simulink model "GenOptRockerMomtryDisHndlr_harness"  (R2017b)
settings: Solver=FixedStepDiscrete  StartTime=0.0  StopTime=0.9  FixedStep=SAMPLE_TIME_CONFIGSET_0p01_S  RelTol=1e-3
undefined symbols (not defined in the file or in its folder): EnCtrlDisSt, EnCtrlSeln, EnCtrlSts, sigbuilder_block
libraries: simulink x1
settings Model: SldvGeneratedHarnessModel=TestUnitModel=temp_GenOptRockerMomtryDisHndlr|  Creator=KIH3CPW  LastModifiedBy=KIH3CPW
settings DataIOCC: SaveOutput=off  SaveTime=off
settings OptimizationCC: DefaultParameterBehavior=Inlined  ZeroExternalMemoryAtStartup=off  ZeroInternalMemoryAtStartup=off  NoFixptDivByZeroProtection=on  EfficientFloat2IntCast=on  LifeSpan=inf
settings DebuggingCC: SignalInfNanChecking=error  SignalRangeChecking=warning  AlgebraicLoopMsg=error  SaveWithDisabledLinksMsg=error  SaveWithParameterizedLinksMsg=error  BlockPriorityViolationMsg=error  SolverPrmCheckMsg=warning  InheritedTsInSrcMsg=none  CheckMatrixSingularityMsg=error  IntegerOverflowMsg=error  ParameterUnderflowMsg=error  ParameterTunabilityLossMsg=error  FixptConstUnderflowMsg=warning  FixptConstOverflowMsg=error  VectorMatrixConversionMsg=warning  SignalLabelMismatchMsg=warning  UnconnectedInputMsg=error  UnconnectedOutputMsg=error  UnconnectedLineMsg=error  SFcnCompatibilityMsg=warning  FrameProcessingCompatibilityMsg=warning  UniqueDataStoreMsg=error  RootOutportRequireBusObject=error  AssertControl=DisableAll  ModelReferenceIOMismatchMessage=warning  UnknownTsInhSupMsg=error  StateNameClashWarn=warning  StrictBusMsg=ErrorOnBusTreatedAsVector  NonBusSignalsTreatedAsBus=warning  IntegerSaturationMsg=error
settings HardwareCC: ProdBitPerPointer=32  ProdBitPerSizeT=32  ProdBitPerPtrDiffT=32  ProdLargestAtomicInteger=Long  ProdLargestAtomicFloat=Double  ProdEndianess=BigEndian  ProdWordSize=32  ProdHWDeviceType=Freescale->32-bit PowerPC
settings ModelReferenceCC: EnableRefExpFcnMdlSchedulingChecks=off  ModelReferencePassRootInputsByReference=off
settings SFSimCC: SimGenImportedTypeDefs=on  MATLABDynamicMemAlloc=off
settings RTWCC: SystemTargetFile=autosar.tlc  GenCodeOnly=on  TemplateMakefile=ert_default_tmf  Description=AUTOSAR  GenerateReport=on  IncludeHyperlinkInReport=on  LaunchReport=on  GenerateTraceInfo=on  GenerateTraceReport=on  GenerateTraceReportSl=on  GenerateTraceReportSf=on  GenerateTraceReportEml=on
settings CodeAppCC: IgnoreCustomStorageClasses=off  MaxIdLength=63  SimulinkDataObjDesc=on  SFDataObjDesc=on  InsertBlockDesc=on  StateflowObjectComments=on  MATLABSourceComments=on
settings STFCustomTargetCC: TargetLangStandard=C99 (ISO)  CodeReplacementLibrary=JD IFL IFX CRL Tables  MultiwordLength=256  ParMdlRefBuildCompliant=on  CompOptLevelCompliant=on  IncludeMdlTerminateFcn=off  CombineOutputUpdateFcns=on  SuppressErrorStatus=on  ERTCustomFileBanners=on  MultiInstanceERTCode=on  CodeInterfacePackaging=Reusable function  SupportNonFinite=off  SupportComplex=off  SupportContinuousTime=off  SupportNonInlinedSFcns=off  RemoveResetFunc=on  ParenthesesLevel=Maximum  MATLABClassNameForMDSCustomization=Simulink.SoftwareTarget.ERTCustomization  AutosarCompliant=on  GRTInterface=off  UseToolchainInfoCompliant=on  LookupTableObjectStructAxisOrder=2,1,3,4,...  LUTObjectStructOrderEvenSpacing=Size,Table,Breakpoints  SystemTargetFile=autosar.tlc
settings ERTTargetCC: TargetLangStandard=C99 (ISO)  CodeReplacementLibrary=JD IFL IFX CRL Tables  ConcurrentExecutionCompliant=off  IncludeMdlTerminateFcn=off  SuppressErrorStatus=on  MultiInstanceERTCode=on  CodeInterfacePackaging=Reusable function  SupportNonFinite=off  SupportComplex=off  ParenthesesLevel=Maximum  ModelStepFunctionPrototypeControlCompliant=off  CPPClassGenCompliant=off  AutosarCompliant=on  LookupTableObjectStructAxisOrder=2,1,3,4,...  LUTObjectStructOrderEvenSpacing=Size,Table,Breakpoints  InlinedParameterPlacement=NonHierarchical  ERTSrcFileBannerTemplate=JD_AUTOSAR_ert_code_template.cgt  ERTHdrFileBannerTemplate=JD_AUTOSAR_ert_code_template.cgt  ERTDataSrcFileTemplate=JD_AUTOSAR_ert_code_template.cgt  ERTDataHdrFileTemplate=JD_AUTOSAR_ert_code_template.cgt  ERTCustomFileTemplate=example_file_process.tlc
settings ConfigComp: CovEnable=on  RecordCoverage=on  CovSaveName=cvdata  CovMetricSettings=dcmw  CovHTMLOptions=on  CovHtmlReporting=on  CovSaveCumulativeToWorkspaceVar=on  CovSaveSingleToWorkspaceVar=on  CovCumulativeReport=on  CovShowResultsExplorer=off  CovReportOnPause=off  CovModelRefEnable=on

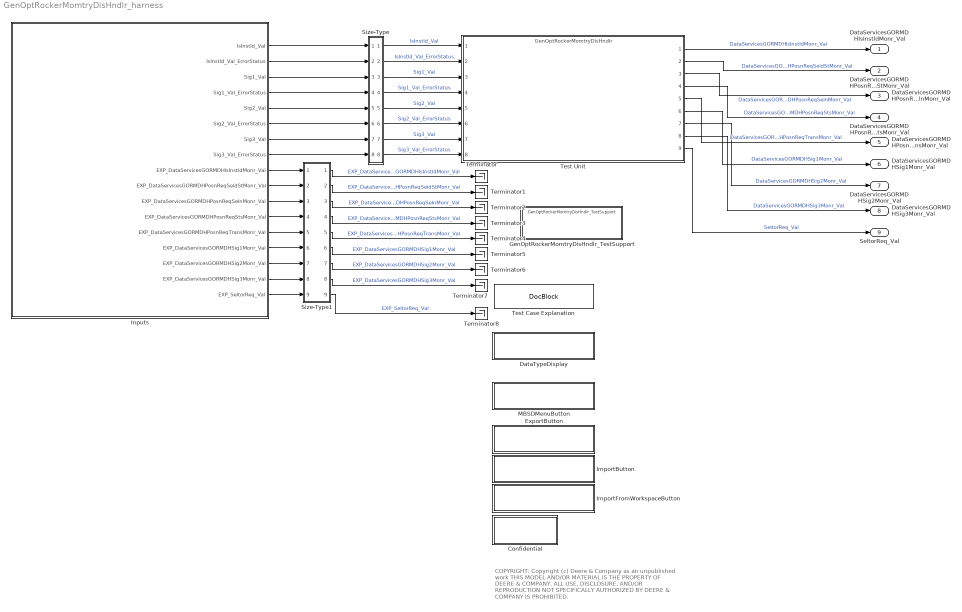
== system GenOptRockerMomtryDisHndlr_harness ==
  note: COPYRIGHT:
      | Copyright (c) Deere & Company as an unpublished work
      | THIS MODEL AND/OR MATERIAL IS THE PROPERTY OF
      | DEERE & COMPANY.  ALL USE, DISCLOSURE, AND/OR
      | REPRODUCTION NOT SPECIFICALLY AUTHORIZED BY
      | DEERE & COMPANY IS PROHIBITED.
  Confidential : Subsystem
      mask Display: image('ConfidentialStamp.jpg')
  DataTypeDisplay : Subsystem  LoadFcn=set_param(gcb,'AttributesFormatString','');  StartFcn=set_param(gcb,'AttributesFormatString','');
      settings: OpenFcn=set_param(gcb,'AttributesFormatString',findModelIDT(gcs));
      mask Display: fprintf(['Double-click to show' char(10) 'Base Data Type'])
  ExportButton : Subsystem  LoadFcn=set_param(gcb,'AttributesFormatString','');  StartFcn=set_param(gcb,'AttributesFormatString','');
      settings: OpenFcn=JD.Model.AddImportExportSwitch.PerformExport(gcs)
      mask Display: fprintf(['Export Data from Signal Builder'])
  GenOptRockerMomtryDisHndlr_TestSupport : ModelReference  ModelNameDialog=GenOptRockerMomtryDisHndlr_TestSupport  SimulationMode=Normal  ModelReferenceVersion=1.1
  ImportButton : Subsystem  LoadFcn=set_param(gcb,'AttributesFormatString','');  StartFcn=set_param(gcb,'AttributesFormatString','');
      settings: OpenFcn=JD.Model.AddImportExportSwitch.PerformImport(gcs)
      mask Display: fprintf(['Import Data to Signal Builder'])
  ImportFromWorkspaceButton : Subsystem  LoadFcn=set_param(gcb,'AttributesFormatString','');  StartFcn=set_param(gcb,'AttributesFormatString','');
      settings: OpenFcn=JD.Model.AddImportExportSwitch.PerformImportfromWorkspace(gcs)
      mask Display: fprintf(['Import Data from Workspace'])
  Inputs : Subsystem  Tag=STV Subsys  LoadFcn=sigbuilder_block('load');  StartFcn=sigbuilder_block('start');  StopFcn=sigbuilder_block('stop');  ClipboardFcn=sigbuilder_block('clipboard');  mask(Sigbuilder block){tuvar=[0:10]}
      mask init:
      | if ~strcmp(get_param(bdroot(gcb),'SimulationStatus'),'stopped'),tuvar = sigbuilder_block('maskInit'); end
      settings: CopyFcn=sigbuilder_block('copy');  DeleteFcn=sigbuilder_block('delete');  ModelCloseFcn=sigbuilder_block('modelClose');  PreSaveFcn=sigbuilder_block('preSave');  PauseFcn=sigbuilder_block('pause');  ContinueFcn=sigbuilder_block('continue');  NameChangeFcn=sigbuilder_block('namechange');  OpenFcn=sigbuilder_block('open',[360.75 33 681.75 578.25 ]);  CloseFcn=sigbuilder_block('close');
      mask Display: plot(0, 0, 100, 100,[2, 2, 32, 32, 2], [68, 8, 8, 68, 68],[32, 2], [38, 38], [32, 19, 2],[53, 60, 44], [32, 17, 17, 2],[16, 16, 31, 31]);txt = getActiveGroup(gcbh);text(2, 100, txt,'verticalAlignment', 'top');
  MBSDMenuButton : Subsystem
      settings: OpenFcn=JD_MBSDMenu
      mask Display: fprintf('MBSD Menu')
  Size-Type : Subsystem
  Size-Type1 : Subsystem
  Terminator{,1..8} (9 alike) : Terminator
  Test Case Explanation : simulink/Model-Wide Utilities/DocBlock  DocumentType=Text
  Test Unit : ModelReference  ModelNameDialog=GenOptRockerMomtryDisHndlr  SimulationMode=Normal  ModelReferenceVersion=1.51
  DataServicesGORMDHIsInstldMonr_Val : Outport  OutDataTypeStr=Enum: DiagBool  PortDimensions=1
  DataServicesGORMDHPosnReqSeldStMonr_Val : Outport  Port=2  OutDataTypeStr=Enum: EnCtrlDisSt  PortDimensions=1
  DataServicesGORMDHPosnReqSelnMonr_Val : Outport  Port=3  OutDataTypeStr=Enum: EnCtrlSeln  PortDimensions=1
  DataServicesGORMDHPosnReqStsMonr_Val : Outport  Port=4  OutDataTypeStr=Enum: EnCtrlSts  PortDimensions=1
  DataServicesGORMDHPosnReqTransMonr_Val : Outport  Port=5  OutDataTypeStr=CntAbsMod  PortDimensions=1
  DataServicesGORMDHSig1Monr_Val : Outport  Port=6  OutDataTypeStr=Enum: DiagBool  PortDimensions=1
  DataServicesGORMDHSig2Monr_Val : Outport  Port=7  OutDataTypeStr=Enum: DiagBool  PortDimensions=1
  DataServicesGORMDHSig3Monr_Val : Outport  Port=8  OutDataTypeStr=Enum: DiagBool  PortDimensions=1
  SeltorReq_Val : Outport  Port=9  OutDataTypeStr=Bus: RecCtrlSelr  PortDimensions=1  BusOutputAsStruct=on
  wires:
  Size-Type/1(Out1) -> Test Unit/1  "IsInstld_Val"
  Size-Type/2(Out2) -> Test Unit/2  "IsInstld_Val_ErrorStatus"
  Size-Type/3(Out3) -> Test Unit/3  "Sig1_Val"
  Size-Type/4(Out4) -> Test Unit/4  "Sig1_Val_ErrorStatus"
  Size-Type/5(Out5) -> Test Unit/5  "Sig2_Val"
  Size-Type/6(Out6) -> Test Unit/6  "Sig2_Val_ErrorStatus"
  Size-Type/7(Out7) -> Test Unit/7  "Sig3_Val"
  Size-Type/8(Out8) -> Test Unit/8  "Sig3_Val_ErrorStatus"
  Test Unit/1 -> DataServicesGORMDHIsInstldMonr_Val/1  "DataServicesGORMDHIsInstldMonr_Val"
  Test Unit/2 -> DataServicesGORMDHPosnReqSeldStMonr_Val/1  "DataServicesGORMDHPosnReqSeldStMonr_Val"
  Test Unit/3 -> DataServicesGORMDHPosnReqSelnMonr_Val/1  "DataServicesGORMDHPosnReqSelnMonr_Val"
  Test Unit/4 -> DataServicesGORMDHPosnReqStsMonr_Val/1  "DataServicesGORMDHPosnReqStsMonr_Val"
  Test Unit/5 -> DataServicesGORMDHPosnReqTransMonr_Val/1  "DataServicesGORMDHPosnReqTransMonr_Val"
  Test Unit/6 -> DataServicesGORMDHSig1Monr_Val/1  "DataServicesGORMDHSig1Monr_Val"
  Test Unit/7 -> DataServicesGORMDHSig2Monr_Val/1  "DataServicesGORMDHSig2Monr_Val"
  Test Unit/8 -> DataServicesGORMDHSig3Monr_Val/1  "DataServicesGORMDHSig3Monr_Val"
  Test Unit/9 -> SeltorReq_Val/1  "SeltorReq_Val"
  Inputs/1(IsInstld_Val) -> Size-Type/1(In1)
  Inputs/2(IsInstld_Val_ErrorStatus) -> Size-Type/2(In2)
  Inputs/3(Sig1_Val) -> Size-Type/3(In3)
  Inputs/4(Sig1_Val_ErrorStatus) -> Size-Type/4(In4)
  Inputs/5(Sig2_Val) -> Size-Type/5(In5)
  Inputs/6(Sig2_Val_ErrorStatus) -> Size-Type/6(In6)
  Inputs/7(Sig3_Val) -> Size-Type/7(In7)
  Inputs/8(Sig3_Val_ErrorStatus) -> Size-Type/8(In8)
  Size-Type1/2(Out2) -> Terminator1/1  "EXP_DataServicesGORMDHPosnReqSeldStMonr_Val"
  Size-Type1/1(Out1) -> Terminator/1  "EXP_DataServicesGORMDHIsInstldMonr_Val"
  Size-Type1/3(Out3) -> Terminator2/1  "EXP_DataServicesGORMDHPosnReqSelnMonr_Val"
  Size-Type1/4(Out4) -> Terminator3/1  "EXP_DataServicesGORMDHPosnReqStsMonr_Val"
  Size-Type1/5(Out5) -> Terminator4/1  "EXP_DataServicesGORMDHPosnReqTransMonr_Val"
  Size-Type1/6(Out6) -> Terminator5/1  "EXP_DataServicesGORMDHSig1Monr_Val"
  Size-Type1/7(Out7) -> Terminator6/1  "EXP_DataServicesGORMDHSig2Monr_Val"
  Size-Type1/8(Out8) -> Terminator7/1  "EXP_DataServicesGORMDHSig3Monr_Val"
  Inputs/9(EXP_DataServicesGORMDHIsInstldMonr_Val) -> Size-Type1/1(In1)
  Inputs/10(EXP_DataServicesGORMDHPosnReqSeldStMonr_Val) -> Size-Type1/2(In2)
  Inputs/11(EXP_DataServicesGORMDHPosnReqSelnMonr_Val) -> Size-Type1/3(In3)
  Inputs/12(EXP_DataServicesGORMDHPosnReqStsMonr_Val) -> Size-Type1/4(In4)
  Inputs/13(EXP_DataServicesGORMDHPosnReqTransMonr_Val) -> Size-Type1/5(In5)
  Inputs/14(EXP_DataServicesGORMDHSig1Monr_Val) -> Size-Type1/6(In6)
  Inputs/15(EXP_DataServicesGORMDHSig2Monr_Val) -> Size-Type1/7(In7)
  Inputs/16(EXP_DataServicesGORMDHSig3Monr_Val) -> Size-Type1/8(In8)
  Inputs/17(EXP_SeltorReq_Val) -> Size-Type1/9(In9)
  Size-Type1/9(Out9) -> Terminator8/1  "EXP_SeltorReq_Val"

== system GenOptRockerMomtryDisHndlr_harness/Confidential ==

== system GenOptRockerMomtryDisHndlr_harness/DataTypeDisplay ==

== system GenOptRockerMomtryDisHndlr_harness/ExportButton ==

== system GenOptRockerMomtryDisHndlr_harness/ImportButton ==

== system GenOptRockerMomtryDisHndlr_harness/ImportFromWorkspaceButton ==

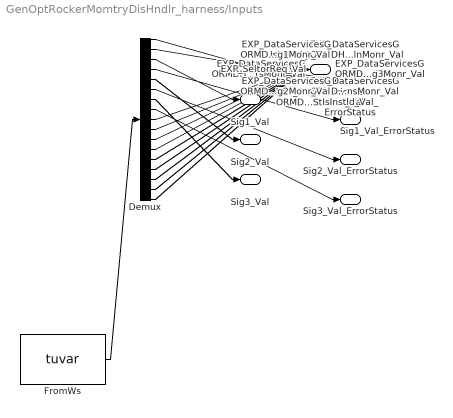
== system GenOptRockerMomtryDisHndlr_harness/Inputs ==
  Demux : Demux  Tag=STV Demux  Outputs=17
  FromWs : FromWorkspace  Tag=STV FromWs  VariableName=tuvar  SampleTime=0
      SigBuilderData=|
      | dataSet(1).timeRange = [0 0.2]
      | dataSet(1).name = 'TP0'
      | dataSet(2).timeRange = [0 1.1]
      | dataSet(2).name = 'TP1'
      | dataSet(3).timeRange = [0 0.4]
      | dataSet(3).name = 'TP2'
      | dataSet(4).timeRange = [0 3.5]
      | dataSet(4).name = 'TP3'
      | dataSet(5).timeRange = [0 0.4]
      | dataSet(5).name = 'TP4'
      | dataSet(6).timeRange = [0 1.4]
      | dataSet(6).name = 'TP5'
      | dataSet(7).timeRange = [0 0.9]
      | dataSet(7).name = 'TP6'
      | sbobj.Name = 'Signal Builder'
      | sbobj.Groups(1).Name = 'TP0'
      | sbobj.Groups(1).Signals(1).Name = 'IsInstld_Val'
      | sbobj.Groups(1).Signals(1).XData = [0 0.1 0.1 0.2]
      | sbobj.Groups(1).Signals(1).YData = [0 0 1 1]
      | sbobj.Groups(1).Signals(2).Name = 'IsInstld_Val_ErrorStatus'
      | sbobj.Groups(1).Signals(2).XData = [0 0.1 0.2]
      | sbobj.Groups(1).Signals(2).YData = [1 1 1]
      | sbobj.Groups(1).Signals(3).Name = 'Sig1_Val'
      | sbobj.Groups(1).Signals(3).XData = [0 0.1 0.2]
      | sbobj.Groups(1).Signals(3).YData = [0 0 0]
      | sbobj.Groups(1).Signals(4).Name = 'Sig1_Val_ErrorStatus'
      | sbobj.Groups(1).Signals(4).XData = [0 0.1 0.1 0.2]
      | sbobj.Groups(1).Signals(4).YData = [0 0 1 1]
      | sbobj.Groups(1).Signals(5).Name = 'Sig2_Val'
      | sbobj.Groups(1).Signals(5).XData = [0 0.1 0.2]
      | sbobj.Groups(1).Signals(5).YData = [0 0 0]
      | sbobj.Groups(1).Signals(6).Name = 'Sig2_Val_ErrorStatus'
      | sbobj.Groups(1).Signals(6).XData = [0 0.1 0.1 0.2]
      | sbobj.Groups(1).Signals(6).YData = [0 0 1 1]
      | sbobj.Groups(1).Signals(7).Name = 'Sig3_Val'
      | sbobj.Groups(1).Signals(7).XData = [0 0.1 0.1 0.2]
      | sbobj.Groups(1).Signals(7).YData = [0 0 1 1]
      | sbobj.Groups(1).Signals(8).Name = 'Sig3_Val_ErrorStatus'
      | sbobj.Groups(1).Signals(8).XData = [0 0.1 0.1 0.2]
      | sbobj.Groups(1).Signals(8).YData = [0 0 1 1]
      | sbobj.Groups(1).Signals(9).Name = 'EXP_DataServicesGORMDHIsInstldMonr_Val'
      | sbobj.Groups(1).Signals(9).XData = [0 0.1 0.1 0.2]
      | sbobj.Groups(1).Signals(9).YData = [0 0 1 1]
      | sbobj.Groups(1).Signals(10).Name = 'EXP_DataServicesGORMDHPosnReqSeldStMonr_Val'
      | sbobj.Groups(1).Signals(10).XData = [0 0.1 0.2]
      | sbobj.Groups(1).Signals(10).YData = [0 0 0]
      | sbobj.Groups(1).Signals(11).Name = 'EXP_DataServicesGORMDHPosnReqSelnMonr_Val'
      | sbobj.Groups(1).Signals(11).XData = [0 0.1 0.2]
      | sbobj.Groups(1).Signals(11).YData = [0 0 0]
      | sbobj.Groups(1).Signals(12).Name = 'EXP_DataServicesGORMDHPosnReqStsMonr_Val'
      | sbobj.Groups(1).Signals(12).XData = [0 0.1 0.1 0.2]
      | sbobj.Groups(1).Signals(12).YData = [5 5 0 0]
      | sbobj.Groups(1).Signals(13).Name = 'EXP_DataServicesGORMDHPosnReqTransMonr_Val'
      | sbobj.Groups(1).Signals(13).XData = [0 0.1 0.2]
      | sbobj.Groups(1).Signals(13).YData = [0 0 0]
      | sbobj.Groups(1).Signals(14).Name = 'EXP_DataServicesGORMDHSig1Monr_Val'
      | sbobj.Groups(1).Signals(14).XData = [0 0.1 0.2]
      | sbobj.Groups(1).Signals(14).YData = [0 0 0]
      | sbobj.Groups(1).Signals(15).Name = 'EXP_DataServicesGORMDHSig2Monr_Val'
      | sbobj.Groups(1).Signals(15).XData = [0 0.1 0.2]
      | sbobj.Groups(1).Signals(15).YData = [0 0 0]
      | sbobj.Groups(1).Signals(16).Name = 'EXP_DataServicesGORMDHSig3Monr_Val'
      | sbobj.Groups(1).Signals(16).XData = [0 0.1 0.1 0.2]
      | sbobj.Groups(1).Signals(16).YData = [0 0 1 1]
      | sbobj.Groups(1).Signals(17).Name = 'EXP_SeltorReq_Val'
      | sbobj.Groups(1).Signals(17).XData = [0 0.1 0.2]
      | sbobj.Groups(1).Signals(17).YData = [0 0 0]
      | sbobj.Groups(1).TimeRange = [0 0.2]
      | sbobj.Groups(2).Name = 'TP1'
      | sbobj.Groups(2).Signals(1).Name = 'IsInstld_Val'
      | sbobj.Groups(2).Signals(1).XData = [0 0.1 0.1 0.2 0.3 0.4 0.5 0.6 0.7 0.8 0.9 1 1.1]
      | sbobj.Groups(2).Signals(1).YData = [0 0 1 1 1 1 1 1 1 1 1 1 1]
      | sbobj.Groups(2).Signals(2).Name = 'IsInstld_Val_ErrorStatus'
      | sbobj.Groups(2).Signals(2).XData = [0 0.1 0.2 0.3 0.4 0.5 0.6 0.7 0.8 0.9 1 1.1]
      | sbobj.Groups(2).Signals(2).YData = [1 1 1 1 1 1 1 1 1 1 1 1]
      | sbobj.Groups(2).Signals(3).Name = 'Sig1_Val'
      | sbobj.Groups(2).Signals(3).XData = [0 0.1 0.2 0.3 0.4 0.5 0.6 0.7 0.7 0.8 0.9 1 1.1]
      | sbobj.Groups(2).Signals(3).YData = [0 0 0 0 0 0 0 0 1 1 1 1 1]
      | sbobj.Groups(2).Signals(4).Name = 'Sig1_Val_ErrorStatus'
      | sbobj.Groups(2).Signals(4).XData = [0 0.1 0.1 0.2 0.3 0.3 0.4 0.5 0.6 0.7 0.7 0.8 0.9 1 1.1]
      | sbobj.Groups(2).Signals(4).YData = [0 0 1 1 1 0 0 0 0 0 1 1 1 1 1]
      | sbobj.Groups(2).Signals(5).Name = 'Sig2_Val'
      | sbobj.Groups(2).Signals(5).XData = [0 0.1 0.2 0.3 0.4 0.5 0.5 0.6 0.7 0.7 0.8 0.9 0.9 1 1.1]
      | sbobj.Groups(2).Signals(5).YData = [0 0 0 0 0 0 1 1 1 0 0 0 1 1 1]
      | sbobj.Groups(2).Signals(6).Name = 'Sig2_Val_ErrorStatus'
      | sbobj.Groups(2).Signals(6).XData = [0 0.1 0.1 0.2 0.3 0.3 0.4 0.5 0.5 0.6 0.7 0.7 0.8 0.9 0.9 1 1.1]
      | sbobj.Groups(2).Signals(6).YData = [0 0 1 1 1 0 0 0 1 1 1 0 0 0 1 1 1]
      | sbobj.Groups(2).Signals(7).Name = 'Sig3_Val'
      | sbobj.Groups(2).Signals(7).XData = [0 0.1 0.1 0.2 0.3 0.3 0.4 0.4 0.5 0.5 0.6 0.6 0.7 0.7 0.8 0.8 0.9 0.9 1 1 1.1]
      | sbobj.Groups(2).Signals(7).YData = [0 0 1 1 1 0 0 1 1 0 0 1 1 0 0 1 1 0 0 1 1]
      | sbobj.Groups(2).Signals(8).Name = 'Sig3_Val_ErrorStatus'
      | sbobj.Groups(2).Signals(8).XData = [0 0.1 0.1 0.2 0.3 0.3 0.4 0.4 0.5 0.5 0.6 0.6 0.7 0.7 0.8 0.8 0.9 0.9 1 1 1.1]
      | sbobj.Groups(2).Signals(8).YData = [0 0 1 1 1 0 0 1 1 0 0 1 1 0 0 1 1 0 0 1 1]
      | sbobj.Groups(2).Signals(9).Name = 'EXP_DataServicesGORMDHIsInstldMonr_Val'
      | sbobj.Groups(2).Signals(9).XData = [0 0.1 0.1 0.2 0.3 0.4 0.5 0.6 0.7 0.8 0.9 1 1.1]
      | sbobj.Groups(2).Signals(9).YData = [0 0 1 1 1 1 1 1 1 1 1 1 1]
      | sbobj.Groups(2).Signals(10).Name = 'EXP_DataServicesGORMDHPosnReqSeldStMonr_Val'
      | sbobj.Groups(2).Signals(10).XData = [0 0.1 0.2 0.3 0.4 0.5 0.6 0.7 0.8 0.9 1 1 1.1]
      | sbobj.Groups(2).Signals(10).YData = [0 0 0 0 0 0 0 0 0 0 0 1 1]
      | sbobj.Groups(2).Signals(11).Name = 'EXP_DataServicesGORMDHPosnReqSelnMonr_Val'
      | sbobj.Groups(2).Signals(11).XData = [0 0.1 0.2 0.3 0.4 0.5 0.6 0.7 0.8 0.9 1 1 1.1]
      | sbobj.Groups(2).Signals(11).YData = [0 0 0 0 0 0 0 0 0 0 0 2 2]
      | sbobj.Groups(2).Signals(12).Name = 'EXP_DataServicesGORMDHPosnReqStsMonr_Val'
      | sbobj.Groups(2).Signals(12).XData = [0 0.1 0.1 0.2 0.3 0.4 0.5 0.6 0.7 0.8 0.9 1 1.1]
      | sbobj.Groups(2).Signals(12).YData = [5 5 0 0 0 0 0 0 0 0 0 0 0]
      | sbobj.Groups(2).Signals(13).Name = 'EXP_DataServicesGORMDHPosnReqTransMonr_Val'
      | sbobj.Groups(2).Signals(13).XData = [0 0.1 0.2 0.3 0.4 0.5 0.6 0.7 0.8 0.9 1 1.1]
      | sbobj.Groups(2).Signals(13).YData = [0 0 0 0 0 0 0 0 0 0 0 0]
      | sbobj.Groups(2).Signals(14).Name = 'EXP_DataServicesGORMDHSig1Monr_Val'
      | sbobj.Groups(2).Signals(14).XData = [0 0.1 0.2 0.3 0.4 0.5 0.6 0.7 0.7 0.8 0.9 1 1.1]
      | sbobj.Groups(2).Signals(14).YData = [0 0 0 0 0 0 0 0 1 1 1 1 1]
      | sbobj.Groups(2).Signals(15).Name = 'EXP_DataServicesGORMDHSig2Monr_Val'
      | sbobj.Groups(2).Signals(15).XData = [0 0.1 0.2 0.3 0.4 0.5 0.5 0.6 0.7 0.7 0.8 0.9 0.9 1 1.1]
      | sbobj.Groups(2).Signals(15).YData = [0 0 0 0 0 0 1 1 1 0 0 0 1 1 1]
      | sbobj.Groups(2).Signals(16).Name = 'EXP_DataServicesGORMDHSig3Monr_Val'
      | sbobj.Groups(2).Signals(16).XData = [0 0.1 0.1 0.2 0.3 0.3 0.4 0.4 0.5 0.5 0.6 0.6 0.7 0.7 0.8 0.8 0.9 0.9 1 1 1.1]
      | sbobj.Groups(2).Signals(16).YData = [0 0 1 1 1 0 0 1 1 0 0 1 1 0 0 1 1 0 0 1 1]
      | sbobj.Groups(2).Signals(17).Name = 'EXP_SeltorReq_Val'
      | sbobj.Groups(2).Signals(17).XData = [0 0.1 0.2 0.3 0.4 0.5 0.6 0.7 0.8 0.9 1 1.1]
      | sbobj.Groups(2).Signals(17).YData = [0 0 0 0 0 0 0 0 0 0 0 0]
      | sbobj.Groups(2).TimeRange = [0 1.1]
      | sbobj.Groups(3).Name = 'TP2'
      | sbobj.Groups(3).Signals(1).Name = 'IsInstld_Val'
      | sbobj.Groups(3).Signals(1).XData = [0 0.1 0.1 0.2 0.3 0.4]
      | sbobj.Groups(3).Signals(1).YData = [0 0 1 1 1 1]
      | sbobj.Groups(3).Signals(2).Name = 'IsInstld_Val_ErrorStatus'
      | sbobj.Groups(3).Signals(2).XData = [0 0.1 0.2 0.3 0.4]
      | sbobj.Groups(3).Signals(2).YData = [1 1 1 1 1]
      | sbobj.Groups(3).Signals(3).Name = 'Sig1_Val'
      | sbobj.Groups(3).Signals(3).XData = [0 0.1 0.1 0.2 0.2 0.3 0.4]
      | sbobj.Groups(3).Signals(3).YData = [0 0 1 1 0 0 0]
      | sbobj.Groups(3).Signals(4).Name = 'Sig1_Val_ErrorStatus'
      | sbobj.Groups(3).Signals(4).XData = [0 0.1 0.1 0.2 0.3 0.4]
      | sbobj.Groups(3).Signals(4).YData = [0 0 1 1 1 1]
      | sbobj.Groups(3).Signals(5).Name = 'Sig2_Val'
      | sbobj.Groups(3).Signals(5).XData = [0 0.1 0.1 0.2 0.2 0.3 0.4]
      | sbobj.Groups(3).Signals(5).YData = [0 0 1 1 0 0 0]
      | sbobj.Groups(3).Signals(6).Name = 'Sig2_Val_ErrorStatus'
      | sbobj.Groups(3).Signals(6).XData = [0 0.1 0.1 0.2 0.3 0.4]
      | sbobj.Groups(3).Signals(6).YData = [0 0 1 1 1 1]
      | sbobj.Groups(3).Signals(7).Name = 'Sig3_Val'
      | sbobj.Groups(3).Signals(7).XData = [0 0.1 0.1 0.2 0.3 0.4]
      | sbobj.Groups(3).Signals(7).YData = [0 0 1 1 1 1]
      | sbobj.Groups(3).Signals(8).Name = 'Sig3_Val_ErrorStatus'
      | sbobj.Groups(3).Signals(8).XData = [0 0.1 0.1 0.2 0.3 0.4]
      | sbobj.Groups(3).Signals(8).YData = [0 0 1 1 1 1]
      | sbobj.Groups(3).Signals(9).Name = 'EXP_DataServicesGORMDHIsInstldMonr_Val'
      | sbobj.Groups(3).Signals(9).XData = [0 0.1 0.1 0.2 0.3 0.4]
      | sbobj.Groups(3).Signals(9).YData = [0 0 1 1 1 1]
      | sbobj.Groups(3).Signals(10).Name = 'EXP_DataServicesGORMDHPosnReqSeldStMonr_Val'
      | sbobj.Groups(3).Signals(10).XData = [0 0.1 0.1 0.2 0.2 0.3 0.4]
      | sbobj.Groups(3).Signals(10).YData = [0 0 1 1 0 0 0]
      | sbobj.Groups(3).Signals(11).Name = 'EXP_DataServicesGORMDHPosnReqSelnMonr_Val'
      | sbobj.Groups(3).Signals(11).XData = [0 0.1 0.1 0.2 0.2 0.3 0.4]
      | sbobj.Groups(3).Signals(11).YData = [0 0 2 2 0 0 0]
      | sbobj.Groups(3).Signals(12).Name = 'EXP_DataServicesGORMDHPosnReqStsMonr_Val'
      | sbobj.Groups(3).Signals(12).XData = [0 0.1 0.1 0.2 0.3 0.4]
      | sbobj.Groups(3).Signals(12).YData = [5 5 0 0 0 0]
      | sbobj.Groups(3).Signals(13).Name = 'EXP_DataServicesGORMDHPosnReqTransMonr_Val'
      | sbobj.Groups(3).Signals(13).XData = [0 0.1 0.2 0.2 0.3 0.4]
      | sbobj.Groups(3).Signals(13).YData = [0 0 0 1 1 1]
      | sbobj.Groups(3).Signals(14).Name = 'EXP_DataServicesGORMDHSig1Monr_Val'
      | sbobj.Groups(3).Signals(14).XData = [0 0.1 0.1 0.2 0.2 0.3 0.4]
      | sbobj.Groups(3).Signals(14).YData = [0 0 1 1 0 0 0]
      | sbobj.Groups(3).Signals(15).Name = 'EXP_DataServicesGORMDHSig2Monr_Val'
      | sbobj.Groups(3).Signals(15).XData = [0 0.1 0.1 0.2 0.2 0.3 0.4]
      | sbobj.Groups(3).Signals(15).YData = [0 0 1 1 0 0 0]
      | sbobj.Groups(3).Signals(16).Name = 'EXP_DataServicesGORMDHSig3Monr_Val'
      | sbobj.Groups(3).Signals(16).XData = [0 0.1 0.1 0.2 0.3 0.4]
      | sbobj.Groups(3).Signals(16).YData = [0 0 1 1 1 1]
      | sbobj.Groups(3).Signals(17).Name = 'EXP_SeltorReq_Val'
      | sbobj.Groups(3).Signals(17).XData = [0 0.1 0.2 0.3 0.4]
      | sbobj.Groups(3).Signals(17).YData = [0 0 0 0 0]
      | sbobj.Groups(3).TimeRange = [0 0.4]
      | sbobj.Groups(4).Name = 'TP3'
      | sbobj.Groups(4).Signals(1).Name = 'IsInstld_Val'
      | sbobj.Groups(4).Signals(1).XData = [0 0.1 0.1 0.2 0.3 0.4 0.5 0.6 0.7 0.8 0.9 1 1.1 1.2 1.3 1.4 1.5 1.6 1.7 1.8 1.9 2 2.1 2.2 2.3 2.4 2.5 2.6 2.7 2.8 2.9 3 3.1 3.2 3.3 3.4 3.5]
      | sbobj.Groups(4).Signals(1).YData = [0 0 1 1 1 1 1 1 1 1 1 1 1 1 1 1 1 1 1 1 1 1 1 1 1 1 1 1 1 1 1 1 1 1 1 1 1]
      | sbobj.Groups(4).Signals(2).Name = 'IsInstld_Val_ErrorStatus'
      | sbobj.Groups(4).Signals(2).XData = [0 0.1 0.2 0.3 0.4 0.5 0.6 0.7 0.8 0.9 1 1.1 1.2 1.3 1.4 1.5 1.6 1.7 1.8 1.9 2 2.1 2.2 2.3 2.4 2.5 2.6 2.7 2.8 2.9 3 3.1 3.2 3.3 3.4 3.5]
      | sbobj.Groups(4).Signals(2).YData = [1 1 1 1 1 1 1 1 1 1 1 1 1 1 1 1 1 1 1 1 1 1 1 1 1 1 1 1 1 1 1 1 1 1 1 1]
      | sbobj.Groups(4).Signals(3).Name = 'Sig1_Val'
      | sbobj.Groups(4).Signals(3).XData = [0 0.1 0.1 0.2 0.3 0.4 0.5 0.6 0.7 0.8 0.9 1 1.1 1.2 1.3 1.4 1.5 1.6 1.7 1.8 1.8 1.9 1.9 2 2.1 2.2 2.3 2.4 2.5 2.6 2.7 2.8 2.9 3 3.1 3.2 3.3 3.4 3.5]
      | sbobj.Groups(4).Signals(3).YData = [0 0 1 1 1 1 1 1 1 1 1 1 1 1 1 1 1 1 1 1 0 0 1 1 1 1 1 1 1 1 1 1 1 1 1 1 1 1 1]
      | sbobj.Groups(4).Signals(4).Name = 'Sig1_Val_ErrorStatus'
      | sbobj.Groups(4).Signals(4).XData = [0 0.1 0.1 0.2 0.3 0.4 0.5 0.6 0.7 0.8 0.9 1 1.1 1.2 1.3 1.4 1.5 1.6 1.7 1.8 1.9 2 2.1 2.2 2.3 2.4 2.5 2.6 2.7 2.8 2.9 3 3.1 3.2 3.3 3.4 3.5]
      | sbobj.Groups(4).Signals(4).YData = [0 0 1 1 1 1 1 1 1 1 1 1 1 1 1 1 1 1 1 1 1 1 1 1 1 1 1 1 1 1 1 1 1 1 1 1 1]
      | sbobj.Groups(4).Signals(5).Name = 'Sig2_Val'
      | sbobj.Groups(4).Signals(5).XData = [0 0.1 0.1 0.2 0.3 0.4 0.5 0.6 0.7 0.8 0.9 1 1.1 1.2 1.3 1.4 1.5 1.6 1.7 1.8 1.8 1.9 2 2.1 2.2 2.3 2.4 2.5 2.6 2.7 2.8 2.9 3 3.1 3.2 3.3 3.4 3.5]
      | sbobj.Groups(4).Signals(5).YData = [0 0 1 1 1 1 1 1 1 1 1 1 1 1 1 1 1 1 1 1 0 0 0 0 0 0 0 0 0 0 0 0 0 0 0 0 0 0]
      | sbobj.Groups(4).Signals(6).Name = 'Sig2_Val_ErrorStatus'
      | sbobj.Groups(4).Signals(6).XData = [0 0.1 0.1 0.2 0.3 0.4 0.5 0.6 0.7 0.8 0.9 1 1.1 1.2 1.3 1.4 1.5 1.6 1.7 1.8 1.9 2 2.1 2.2 2.3 2.4 2.5 2.6 2.6 2.7 2.7 2.8 2.9 3 3.1 3.2 3.3 3.4 3.5]
      | sbobj.Groups(4).Signals(6).YData = [0 0 1 1 1 1 1 1 1 1 1 1 1 1 1 1 1 1 1 1 1 1 1 1 1 1 1 1 4 4 1 1 1 1 1 1 1 1 1]
      | sbobj.Groups(4).Signals(7).Name = 'Sig3_Val'
      | sbobj.Groups(4).Signals(7).XData = [0 0.1 0.1 0.2 0.3 0.4 0.5 0.6 0.7 0.8 0.9 1 1.1 1.2 1.3 1.4 1.5 1.6 1.7 1.8 1.9 1.9 2 2.1 2.2 2.3 2.4 2.5 2.6 2.7 2.8 2.9 3 3.1 3.2 3.3 3.4 3.5]
      | sbobj.Groups(4).Signals(7).YData = [0 0 1 1 1 1 1 1 1 1 1 1 1 1 1 1 1 1 1 1 1 0 0 0 0 0 0 0 0 0 0 0 0 0 0 0 0 0]
      | sbobj.Groups(4).Signals(8).Name = 'Sig3_Val_ErrorStatus'
      | sbobj.Groups(4).Signals(8).XData = [0 0.1 0.1 0.2 0.3 0.4 0.5 0.6 0.7 0.8 0.9 1 1.1 1.2 1.3 1.4 1.5 1.6 1.7 1.8 1.9 2 2.1 2.2 2.3 2.4 2.5 2.6 2.7 2.8 2.9 3 3.1 3.2 3.3 3.4 3.5]
      | sbobj.Groups(4).Signals(8).YData = [0 0 1 1 1 1 1 1 1 1 1 1 1 1 1 1 1 1 1 1 1 1 1 1 1 1 1 1 1 1 1 1 1 1 1 1 1]
      | sbobj.Groups(4).Signals(9).Name = 'EXP_DataServicesGORMDHIsInstldMonr_Val'
      | sbobj.Groups(4).Signals(9).XData = [0 0.1 0.1 0.2 0.3 0.4 0.5 0.6 0.7 0.8 0.9 1 1.1 1.2 1.3 1.4 1.5 1.6 1.7 1.8 1.9 2 2.1 2.2 2.3 2.4 2.5 2.6 2.7 2.8 2.9 3 3.1 3.2 3.3 3.4 3.5]
      | sbobj.Groups(4).Signals(9).YData = [0 0 1 1 1 1 1 1 1 1 1 1 1 1 1 1 1 1 1 1 1 1 1 1 1 1 1 1 1 1 1 1 1 1 1 1 1]
      | sbobj.Groups(4).Signals(10).Name = 'EXP_DataServicesGORMDHPosnReqSeldStMonr_Val'
      | sbobj.Groups(4).Signals(10).XData = [0 0.1 0.1 0.2 0.3 0.4 0.5 0.6 0.7 0.7 0.8 0.9 1 1.1 1.2 1.3 1.4 1.5 1.6 1.6 1.7 1.8 1.8 1.9 1.9 2 2.1 2.2 2.3 2.4 2.5 2.5 2.6 2.7 2.8 2.9 3 3.1 3.2 3.3 3.4 3.4 3.5]
      | sbobj.Groups(4).Signals(10).YData = [0 0 1 1 1 1 1 1 1 2 2 2 2 2 2 2 2 2 2 3 3 3 0 0 1 1 1 1 1 1 1 2 2 2 2 2 2 2 2 2 2 3 3]
      | sbobj.Groups(4).Signals(11).Name = 'EXP_DataServicesGORMDHPosnReqSelnMonr_Val'
      | sbobj.Groups(4).Signals(11).XData = [0 0.1 0.1 0.2 0.3 0.4 0.5 0.6 0.7 0.8 0.9 1 1.1 1.2 1.3 1.4 1.5 1.6 1.7 1.8 1.8 1.9 1.9 2 2.1 2.2 2.3 2.4 2.5 2.6 2.7 2.8 2.9 3 3.1 3.2 3.3 3.4 3.5]
      | sbobj.Groups(4).Signals(11).YData = [0 0 2 2 2 2 2 2 2 2 2 2 2 2 2 2 2 2 2 2 0 0 3 3 3 3 3 3 3 3 3 3 3 3 3 3 3 3 3]
      | sbobj.Groups(4).Signals(12).Name = 'EXP_DataServicesGORMDHPosnReqStsMonr_Val'
      | sbobj.Groups(4).Signals(12).XData = [0 0.1 0.1 0.2 0.3 0.4 0.5 0.6 0.7 0.8 0.9 1 1.1 1.2 1.3 1.4 1.5 1.6 1.7 1.8 1.9 2 2.1 2.2 2.3 2.4 2.5 2.6 2.7 2.8 2.9 3 3.1 3.2 3.3 3.4 3.5]
      | sbobj.Groups(4).Signals(12).YData = [5 5 0 0 0 0 0 0 0 0 0 0 0 0 0 0 0 0 0 0 0 0 0 0 0 0 0 0 0 0 0 0 0 0 0 0 0]
      | sbobj.Groups(4).Signals(13).Name = 'EXP_DataServicesGORMDHPosnReqTransMonr_Val'
      | sbobj.Groups(4).Signals(13).XData = [0 0.1 0.2 0.3 0.4 0.5 0.6 0.7 0.8 0.9 1 1.1 1.2 1.3 1.4 1.5 1.6 1.7 1.8 1.8 1.9 2 2.1 2.2 2.3 2.4 2.5 2.6 2.7 2.8 2.9 3 3.1 3.2 3.3 3.4 3.5]
      | sbobj.Groups(4).Signals(13).YData = [0 0 0 0 0 0 0 0 0 0 0 0 0 0 0 0 0 0 0 1 1 1 1 1 1 1 1 1 1 1 1 1 1 1 1 1 1]
      | sbobj.Groups(4).Signals(14).Name = 'EXP_DataServicesGORMDHSig1Monr_Val'
      | sbobj.Groups(4).Signals(14).XData = [0 0.1 0.1 0.2 0.3 0.4 0.5 0.6 0.7 0.8 0.9 1 1.1 1.2 1.3 1.4 1.5 1.6 1.7 1.8 1.8 1.9 1.9 2 2.1 2.2 2.3 2.4 2.5 2.6 2.7 2.8 2.9 3 3.1 3.2 3.3 3.4 3.5]
      | sbobj.Groups(4).Signals(14).YData = [0 0 1 1 1 1 1 1 1 1 1 1 1 1 1 1 1 1 1 1 0 0 1 1 1 1 1 1 1 1 1 1 1 1 1 1 1 1 1]
      | sbobj.Groups(4).Signals(15).Name = 'EXP_DataServicesGORMDHSig2Monr_Val'
      | sbobj.Groups(4).Signals(15).XData = [0 0.1 0.1 0.2 0.3 0.4 0.5 0.6 0.7 0.8 0.9 1 1.1 1.2 1.3 1.4 1.5 1.6 1.7 1.8 1.8 1.9 2 2.1 2.2 2.3 2.4 2.5 2.6 2.7 2.8 2.9 3 3.1 3.2 3.3 3.4 3.5]
      | sbobj.Groups(4).Signals(15).YData = [0 0 1 1 1 1 1 1 1 1 1 1 1 1 1 1 1 1 1 1 0 0 0 0 0 0 0 0 0 0 0 0 0 0 0 0 0 0]
      | sbobj.Groups(4).Signals(16).Name = 'EXP_DataServicesGORMDHSig3Monr_Val'
      | sbobj.Groups(4).Signals(16).XData = [0 0.1 0.1 0.2 0.3 0.4 0.5 0.6 0.7 0.8 0.9 1 1.1 1.2 1.3 1.4 1.5 1.6 1.7 1.8 1.9 1.9 2 2.1 2.2 2.3 2.4 2.5 2.6 2.7 2.8 2.9 3 3.1 3.2 3.3 3.4 3.5]
      | sbobj.Groups(4).Signals(16).YData = [0 0 1 1 1 1 1 1 1 1 1 1 1 1 1 1 1 1 1 1 1 0 0 0 0 0 0 0 0 0 0 0 0 0 0 0 0 0]
      | sbobj.Groups(4).Signals(17).Name = 'EXP_SeltorReq_Val'
      | sbobj.Groups(4).Signals(17).XData = [0 0.1 0.2 0.3 0.4 0.5 0.6 0.7 0.8 0.9 1 1.1 1.2 1.3 1.4 1.5 1.6 1.7 1.8 1.9 2 2.1 2.2 2.3 2.4 2.5 2.6 2.7 2.8 2.9 3 3.1 3.2 3.3 3.4 3.5]
      | sbobj.Groups(4).Signals(17).YData = [0 0 0 0 0 0 0 0 0 0 0 0 0 0 0 0 0 0 0 0 0 0 0 0 0 0 0 0 0 0 0 0 0 0 0 0]
      | sbobj.Groups(4).TimeRange = [0 3.5]
      | sbobj.Groups(5).Name = 'TP4'
      | sbobj.Groups(5).Signals(1).Name = 'IsInstld_Val'
      | sbobj.Groups(5).Signals(1).XData = [0 0.1 0.1 0.2 0.3 0.4]
      | sbobj.Groups(5).Signals(1).YData = [0 0 1 1 1 1]
      | sbobj.Groups(5).Signals(2).Name = 'IsInstld_Val_ErrorStatus'
      | sbobj.Groups(5).Signals(2).XData = [0 0.1 0.2 0.3 0.4]
      | sbobj.Groups(5).Signals(2).YData = [1 1 1 1 1]
      | sbobj.Groups(5).Signals(3).Name = 'Sig1_Val'
      | sbobj.Groups(5).Signals(3).XData = [0 0.1 0.2 0.2 0.3 0.4]
      | sbobj.Groups(5).Signals(3).YData = [0 0 0 1 1 1]
      | sbobj.Groups(5).Signals(4).Name = 'Sig1_Val_ErrorStatus'
      | sbobj.Groups(5).Signals(4).XData = [0 0.1 0.1 0.2 0.3 0.4]
      | sbobj.Groups(5).Signals(4).YData = [0 0 1 1 1 1]
      | sbobj.Groups(5).Signals(5).Name = 'Sig2_Val'
      | sbobj.Groups(5).Signals(5).XData = [0 0.1 0.2 0.2 0.3 0.3 0.4]
      | sbobj.Groups(5).Signals(5).YData = [0 0 0 1 1 0 0]
      | sbobj.Groups(5).Signals(6).Name = 'Sig2_Val_ErrorStatus'
      | sbobj.Groups(5).Signals(6).XData = [0 0.1 0.1 0.2 0.3 0.4]
      | sbobj.Groups(5).Signals(6).YData = [0 0 1 1 1 1]
      | sbobj.Groups(5).Signals(7).Name = 'Sig3_Val'
      | sbobj.Groups(5).Signals(7).XData = [0 0.1 0.1 0.2 0.3 0.3 0.4]
      | sbobj.Groups(5).Signals(7).YData = [0 0 1 1 1 0 0]
      | sbobj.Groups(5).Signals(8).Name = 'Sig3_Val_ErrorStatus'
      | sbobj.Groups(5).Signals(8).XData = [0 0.1 0.1 0.2 0.3 0.4]
      | sbobj.Groups(5).Signals(8).YData = [0 0 1 1 1 1]
      | sbobj.Groups(5).Signals(9).Name = 'EXP_DataServicesGORMDHIsInstldMonr_Val'
      | sbobj.Groups(5).Signals(9).XData = [0 0.1 0.1 0.2 0.3 0.4]
      | sbobj.Groups(5).Signals(9).YData = [0 0 1 1 1 1]
      | sbobj.Groups(5).Signals(10).Name = 'EXP_DataServicesGORMDHPosnReqSeldStMonr_Val'
      | sbobj.Groups(5).Signals(10).XData = [0 0.1 0.2 0.2 0.3 0.4]
      | sbobj.Groups(5).Signals(10).YData = [0 0 0 1 1 1]
      | sbobj.Groups(5).Signals(11).Name = 'EXP_DataServicesGORMDHPosnReqSelnMonr_Val'
      | sbobj.Groups(5).Signals(11).XData = [0 0.1 0.2 0.2 0.3 0.3 0.4]
      | sbobj.Groups(5).Signals(11).YData = [0 0 0 2 2 3 3]
      | sbobj.Groups(5).Signals(12).Name = 'EXP_DataServicesGORMDHPosnReqStsMonr_Val'
      | sbobj.Groups(5).Signals(12).XData = [0 0.1 0.1 0.2 0.3 0.4]
      | sbobj.Groups(5).Signals(12).YData = [5 5 0 0 0 0]
      | sbobj.Groups(5).Signals(13).Name = 'EXP_DataServicesGORMDHPosnReqTransMonr_Val'
      | sbobj.Groups(5).Signals(13).XData = [0 0.1 0.2 0.3 0.4]
      | sbobj.Groups(5).Signals(13).YData = [0 0 0 0 0]
      | sbobj.Groups(5).Signals(14).Name = 'EXP_DataServicesGORMDHSig1Monr_Val'
      | sbobj.Groups(5).Signals(14).XData = [0 0.1 0.2 0.2 0.3 0.4]
      | sbobj.Groups(5).Signals(14).YData = [0 0 0 1 1 1]
      | sbobj.Groups(5).Signals(15).Name = 'EXP_DataServicesGORMDHSig2Monr_Val'
      | sbobj.Groups(5).Signals(15).XData = [0 0.1 0.2 0.2 0.3 0.3 0.4]
      | sbobj.Groups(5).Signals(15).YData = [0 0 0 1 1 0 0]
      | sbobj.Groups(5).Signals(16).Name = 'EXP_DataServicesGORMDHSig3Monr_Val'
      | sbobj.Groups(5).Signals(16).XData = [0 0.1 0.1 0.2 0.3 0.3 0.4]
      | sbobj.Groups(5).Signals(16).YData = [0 0 1 1 1 0 0]
      | sbobj.Groups(5).Signals(17).Name = 'EXP_SeltorReq_Val'
      | sbobj.Groups(5).Signals(17).XData = [0 0.1 0.2 0.3 0.4]
      | sbobj.Groups(5).Signals(17).YData = [0 0 0 0 0]
      | sbobj.Groups(5).TimeRange = [0 0.4]
      | sbobj.Groups(6).Name = 'TP5'
      | sbobj.Groups(6).Signals(1).Name = 'IsInstld_Val'
      | sbobj.Groups(6).Signals(1).XData = [0 0.1 0.1 0.2 0.3 0.4 0.5 0.6 0.7 0.8 0.9 1 1.1 1.2 1.3 1.4]
      | sbobj.Groups(6).Signals(1).YData = [0 0 1 1 1 1 1 1 1 1 1 1 1 1 1 1]
      | sbobj.Groups(6).Signals(2).Name = 'IsInstld_Val_ErrorStatus'
      | sbobj.Groups(6).Signals(2).XData = [0 0.1 0.2 0.3 0.4 0.5 0.6 0.7 0.8 0.9 1 1.1 1.1 1.2 1.2 1.3 1.3 1.4]
      | sbobj.Groups(6).Signals(2).YData = [1 1 1 1 1 1 1 1 1 1 1 1 2 2 3 3 4 4]
      | sbobj.Groups(6).Signals(3).Name = 'Sig1_Val'
      | sbobj.Groups(6).Signals(3).XData = [0 0.1 0.2 0.3 0.4 0.5 0.6 0.7 0.8 0.9 1 1.1 1.2 1.3 1.4]
      | sbobj.Groups(6).Signals(3).YData = [0 0 0 0 0 0 0 0 0 0 0 0 0 0 0]
      | sbobj.Groups(6).Signals(4).Name = 'Sig1_Val_ErrorStatus'
      | sbobj.Groups(6).Signals(4).XData = [0 0.1 0.1 0.2 0.3 0.4 0.5 0.6 0.7 0.8 0.9 1 1.1 1.1 1.2 1.2 1.3 1.3 1.4]
      | sbobj.Groups(6).Signals(4).YData = [0 0 1 1 1 1 1 1 1 1 1 1 1 2 2 3 3 4 4]
      | sbobj.Groups(6).Signals(5).Name = 'Sig2_Val'
      | sbobj.Groups(6).Signals(5).XData = [0 0.1 0.2 0.3 0.4 0.5 0.6 0.7 0.8 0.9 1 1.1 1.2 1.3 1.4]
      | sbobj.Groups(6).Signals(5).YData = [0 0 0 0 0 0 0 0 0 0 0 0 0 0 0]
      | sbobj.Groups(6).Signals(6).Name = 'Sig2_Val_ErrorStatus'
      | sbobj.Groups(6).Signals(6).XData = [0 0.1 0.1 0.2 0.3 0.4 0.5 0.6 0.7 0.8 0.9 1 1.1 1.1 1.2 1.2 1.3 1.3 1.4]
      | sbobj.Groups(6).Signals(6).YData = [0 0 1 1 1 1 1 1 1 1 1 1 1 2 2 3 3 4 4]
      | sbobj.Groups(6).Signals(7).Name = 'Sig3_Val'
      | sbobj.Groups(6).Signals(7).XData = [0 0.1 0.1 0.2 0.2 0.3 0.4 0.5 0.6 0.7 0.8 0.9 1 1.1 1.2 1.3 1.4]
      | sbobj.Groups(6).Signals(7).YData = [0 0 1 1 0 0 0 0 0 0 0 0 0 0 0 0 0]
      | sbobj.Groups(6).Signals(8).Name = 'Sig3_Val_ErrorStatus'
      | sbobj.Groups(6).Signals(8).XData = [0 0.1 0.1 0.2 0.3 0.4 0.5 0.6 0.7 0.8 0.9 1 1.1 1.1 1.2 1.2 1.3 1.3 1.4]
      | sbobj.Groups(6).Signals(8).YData = [0 0 1 1 1 1 1 1 1 1 1 1 1 2 2 3 3 4 4]
      | sbobj.Groups(6).Signals(9).Name = 'EXP_DataServicesGORMDHIsInstldMonr_Val'
      | sbobj.Groups(6).Signals(9).XData = [0 0.1 0.1 0.2 0.3 0.4 0.5 0.6 0.7 0.8 0.9 1 1.1 1.2 1.3 1.4]
      | sbobj.Groups(6).Signals(9).YData = [0 0 1 1 1 1 1 1 1 1 1 1 1 1 1 1]
      | sbobj.Groups(6).Signals(10).Name = 'EXP_DataServicesGORMDHPosnReqSeldStMonr_Val'
      | sbobj.Groups(6).Signals(10).XData = [0 0.1 0.2 0.3 0.4 0.5 0.6 0.7 0.8 0.9 1 1.1 1.2 1.3 1.4]
      | sbobj.Groups(6).Signals(10).YData = [0 0 0 0 0 0 0 0 0 0 0 0 0 0 0]
      | sbobj.Groups(6).Signals(11).Name = 'EXP_DataServicesGORMDHPosnReqSelnMonr_Val'
      | sbobj.Groups(6).Signals(11).XData = [0 0.1 0.2 0.3 0.4 0.5 0.6 0.7 0.8 0.9 1 1.1 1.2 1.3 1.4]
      | sbobj.Groups(6).Signals(11).YData = [0 0 0 0 0 0 0 0 0 0 0 0 0 0 0]
      | sbobj.Groups(6).Signals(12).Name = 'EXP_DataServicesGORMDHPosnReqStsMonr_Val'
      | sbobj.Groups(6).Signals(12).XData = [0 0.1 0.1 0.2 0.3 0.4 0.5 0.6 0.7 0.8 0.9 1 1.1 1.1 1.2 1.3 1.4]
      | sbobj.Groups(6).Signals(12).YData = [5 5 0 0 0 0 0 0 0 0 0 0 0 6 6 6 6]
      | sbobj.Groups(6).Signals(13).Name = 'EXP_DataServicesGORMDHPosnReqTransMonr_Val'
      | sbobj.Groups(6).Signals(13).XData = [0 0.1 0.2 0.3 0.4 0.5 0.6 0.7 0.8 0.9 1 1.1 1.2 1.3 1.4]
      | sbobj.Groups(6).Signals(13).YData = [0 0 0 0 0 0 0 0 0 0 0 0 0 0 0]
      | sbobj.Groups(6).Signals(14).Name = 'EXP_DataServicesGORMDHSig1Monr_Val'
      | sbobj.Groups(6).Signals(14).XData = [0 0.1 0.2 0.3 0.4 0.5 0.6 0.7 0.8 0.9 1 1.1 1.2 1.3 1.4]
      | sbobj.Groups(6).Signals(14).YData = [0 0 0 0 0 0 0 0 0 0 0 0 0 0 0]
      | sbobj.Groups(6).Signals(15).Name = 'EXP_DataServicesGORMDHSig2Monr_Val'
      | sbobj.Groups(6).Signals(15).XData = [0 0.1 0.2 0.3 0.4 0.5 0.6 0.7 0.8 0.9 1 1.1 1.2 1.3 1.4]
      | sbobj.Groups(6).Signals(15).YData = [0 0 0 0 0 0 0 0 0 0 0 0 0 0 0]
      | sbobj.Groups(6).Signals(16).Name = 'EXP_DataServicesGORMDHSig3Monr_Val'
      | sbobj.Groups(6).Signals(16).XData = [0 0.1 0.1 0.2 0.2 0.3 0.4 0.5 0.6 0.7 0.8 0.9 1 1.1 1.2 1.3 1.4]
      | sbobj.Groups(6).Signals(16).YData = [0 0 1 1 0 0 0 0 0 0 0 0 0 0 0 0 0]
      | sbobj.Groups(6).Signals(17).Name = 'EXP_SeltorReq_Val'
      | sbobj.Groups(6).Signals(17).XData = [0 0.1 0.2 0.3 0.4 0.5 0.6 0.7 0.8 0.9 1 1.1 1.2 1.3 1.4]
      | sbobj.Groups(6).Signals(17).YData = [0 0 0 0 0 0 0 0 0 0 0 0 0 0 0]
      | sbobj.Groups(6).TimeRange = [0 1.4]
      | sbobj.Groups(7).Name = 'TP6'
      | sbobj.Groups(7).Signals(1).Name = 'IsInstld_Val'
      | sbobj.Groups(7).Signals(1).XData = [0 0.1 0.2 0.3 0.4 0.5 0.6 0.7 0.8 0.9]
      | sbobj.Groups(7).Signals(1).YData = [0 0 0 0 0 0 0 0 0 0]
      | sbobj.Groups(7).Signals(2).Name = 'IsInstld_Val_ErrorStatus'
      | sbobj.Groups(7).Signals(2).XData = [0 0.1 0.2 0.3 0.4 0.5 0.6 0.7 0.8 0.9]
      | sbobj.Groups(7).Signals(2).YData = [1 1 1 1 1 1 1 1 1 1]
      | sbobj.Groups(7).Signals(3).Name = 'Sig1_Val'
      | sbobj.Groups(7).Signals(3).XData = [0 0.1 0.2 0.3 0.4 0.5 0.5 0.6 0.7 0.8 0.9]
      | sbobj.Groups(7).Signals(3).YData = [0 0 0 0 0 0 1 1 1 1 1]
      | sbobj.Groups(7).Signals(4).Name = 'Sig1_Val_ErrorStatus'
      | sbobj.Groups(7).Signals(4).XData = [0 0.1 0.1 0.2 0.3 0.4 0.5 0.6 0.7 0.8 0.9]
      | sbobj.Groups(7).Signals(4).YData = [0 0 1 1 1 1 1 1 1 1 1]
      | sbobj.Groups(7).Signals(5).Name = 'Sig2_Val'
      | sbobj.Groups(7).Signals(5).XData = [0 0.1 0.2 0.3 0.3 0.4 0.5 0.5 0.6 0.7 0.7 0.8 0.9]
      | sbobj.Groups(7).Signals(5).YData = [0 0 0 0 1 1 1 0 0 0 1 1 1]
      | sbobj.Groups(7).Signals(6).Name = 'Sig2_Val_ErrorStatus'
      | sbobj.Groups(7).Signals(6).XData = [0 0.1 0.1 0.2 0.3 0.4 0.5 0.6 0.7 0.8 0.9]
      | sbobj.Groups(7).Signals(6).YData = [0 0 1 1 1 1 1 1 1 1 1]
      | sbobj.Groups(7).Signals(7).Name = 'Sig3_Val'
      | sbobj.Groups(7).Signals(7).XData = [0 0.1 0.2 0.2 0.3 0.3 0.4 0.4 0.5 0.5 0.6 0.6 0.7 0.7 0.8 0.8 0.9]
      | sbobj.Groups(7).Signals(7).YData = [0 0 0 1 1 0 0 1 1 0 0 1 1 0 0 1 1]
      | sbobj.Groups(7).Signals(8).Name = 'Sig3_Val_ErrorStatus'
      | sbobj.Groups(7).Signals(8).XData = [0 0.1 0.1 0.2 0.3 0.4 0.5 0.6 0.7 0.8 0.9]
      | sbobj.Groups(7).Signals(8).YData = [0 0 1 1 1 1 1 1 1 1 1]
      | sbobj.Groups(7).Signals(9).Name = 'EXP_DataServicesGORMDHIsInstldMonr_Val'
      | sbobj.Groups(7).Signals(9).XData = [0 0.1 0.2 0.3 0.4 0.5 0.6 0.7 0.8 0.9]
      | sbobj.Groups(7).Signals(9).YData = [0 0 0 0 0 0 0 0 0 0]
      | sbobj.Groups(7).Signals(10).Name = 'EXP_DataServicesGORMDHPosnReqSeldStMonr_Val'
      | sbobj.Groups(7).Signals(10).XData = [0 0.1 0.2 0.3 0.4 0.5 0.6 0.7 0.8 0.9]
      | sbobj.Groups(7).Signals(10).YData = [0 0 0 0 0 0 0 0 0 0]
      | sbobj.Groups(7).Signals(11).Name = 'EXP_DataServicesGORMDHPosnReqSelnMonr_Val'
      | sbobj.Groups(7).Signals(11).XData = [0 0.1 0.2 0.3 0.4 0.5 0.6 0.7 0.8 0.9]
      | sbobj.Groups(7).Signals(11).YData = [0 0 0 0 0 0 0 0 0 0]
      | sbobj.Groups(7).Signals(12).Name = 'EXP_DataServicesGORMDHPosnReqStsMonr_Val'
      | sbobj.Groups(7).Signals(12).XData = [0 0.1 0.2 0.3 0.4 0.5 0.6 0.7 0.8 0.9]
      | sbobj.Groups(7).Signals(12).YData = [5 5 5 5 5 5 5 5 5 5]
      | sbobj.Groups(7).Signals(13).Name = 'EXP_DataServicesGORMDHPosnReqTransMonr_Val'
      | sbobj.Groups(7).Signals(13).XData = [0 0.1 0.2 0.3 0.4 0.5 0.6 0.7 0.8 0.9]
      | sbobj.Groups(7).Signals(13).YData = [0 0 0 0 0 0 0 0 0 0]
      | sbobj.Groups(7).Signals(14).Name = 'EXP_DataServicesGORMDHSig1Monr_Val'
      | sbobj.Groups(7).Signals(14).XData = [0 0.1 0.1 0.2 0.3 0.4 0.5 0.6 0.7 0.8 0.9]
      | sbobj.Groups(7).Signals(14).YData = [0 0 1 1 1 1 1 1 1 1 1]
      | sbobj.Groups(7).Signals(15).Name = 'EXP_DataServicesGORMDHSig2Monr_Val'
      | sbobj.Groups(7).Signals(15).XData = [0 0.1 0.1 0.2 0.3 0.4 0.5 0.6 0.7 0.8 0.9]
      | sbobj.Groups(7).Signals(15).YData = [0 0 1 1 1 1 1 1 1 1 1]
      | sbobj.Groups(7).Signals(16).Name = 'EXP_DataServicesGORMDHSig3Monr_Val'
      | sbobj.Groups(7).Signals(16).XData = [0 0.1 0.1 0.2 0.3 0.4 0.5 0.6 0.7 0.8 0.9]
      | sbobj.Groups(7).Signals(16).YData = [0 0 1 1 1 1 1 1 1 1 1]
      | sbobj.Groups(7).Signals(17).Name = 'EXP_SeltorReq_Val'
      | sbobj.Groups(7).Signals(17).XData = [0 0.1 0.2 0.3 0.4 0.5 0.6 0.7 0.8 0.9]
      | sbobj.Groups(7).Signals(17).YData = [0 0 0 0 0 0 0 0 0 0]
      | sbobj.Groups(7).TimeRange = [0 0.9]
  IsInstld_Val : Outport  Tag=STV Outport
  IsInstld_Val_ErrorStatus : Outport  Tag=STV Outport  Port=2
  Sig1_Val : Outport  Tag=STV Outport  Port=3
  Sig1_Val_ErrorStatus : Outport  Tag=STV Outport  Port=4
  Sig2_Val : Outport  Tag=STV Outport  Port=5
  Sig2_Val_ErrorStatus : Outport  Tag=STV Outport  Port=6
  Sig3_Val : Outport  Tag=STV Outport  Port=7
  Sig3_Val_ErrorStatus : Outport  Tag=STV Outport  Port=8
  EXP_DataServicesGORMDHIsInstldMonr_Val : Outport  Tag=STV Outport  Port=9
  EXP_DataServicesGORMDHPosnReqSeldStMonr_Val : Outport  Tag=STV Outport  Port=10
  EXP_DataServicesGORMDHPosnReqSelnMonr_Val : Outport  Tag=STV Outport  Port=11
  EXP_DataServicesGORMDHPosnReqStsMonr_Val : Outport  Tag=STV Outport  Port=12
  EXP_DataServicesGORMDHPosnReqTransMonr_Val : Outport  Tag=STV Outport  Port=13
  EXP_DataServicesGORMDHSig1Monr_Val : Outport  Tag=STV Outport  Port=14
  EXP_DataServicesGORMDHSig2Monr_Val : Outport  Tag=STV Outport  Port=15
  EXP_DataServicesGORMDHSig3Monr_Val : Outport  Tag=STV Outport  Port=16
  EXP_SeltorReq_Val : Outport  Tag=STV Outport  Port=17
  wires:
  Demux/1 -> IsInstld_Val/1
  Demux/2 -> IsInstld_Val_ErrorStatus/1
  Demux/3 -> Sig1_Val/1
  Demux/4 -> Sig1_Val_ErrorStatus/1
  Demux/5 -> Sig2_Val/1
  Demux/6 -> Sig2_Val_ErrorStatus/1
  Demux/7 -> Sig3_Val/1
  Demux/8 -> Sig3_Val_ErrorStatus/1
  Demux/9 -> EXP_DataServicesGORMDHIsInstldMonr_Val/1
  Demux/10 -> EXP_DataServicesGORMDHPosnReqSeldStMonr_Val/1
  Demux/11 -> EXP_DataServicesGORMDHPosnReqSelnMonr_Val/1
  Demux/12 -> EXP_DataServicesGORMDHPosnReqStsMonr_Val/1
  Demux/13 -> EXP_DataServicesGORMDHPosnReqTransMonr_Val/1
  Demux/14 -> EXP_DataServicesGORMDHSig1Monr_Val/1
  Demux/15 -> EXP_DataServicesGORMDHSig2Monr_Val/1
  Demux/16 -> EXP_DataServicesGORMDHSig3Monr_Val/1
  Demux/17 -> EXP_SeltorReq_Val/1
  FromWs/1 -> Demux/1

== system GenOptRockerMomtryDisHndlr_harness/MBSDMenuButton ==

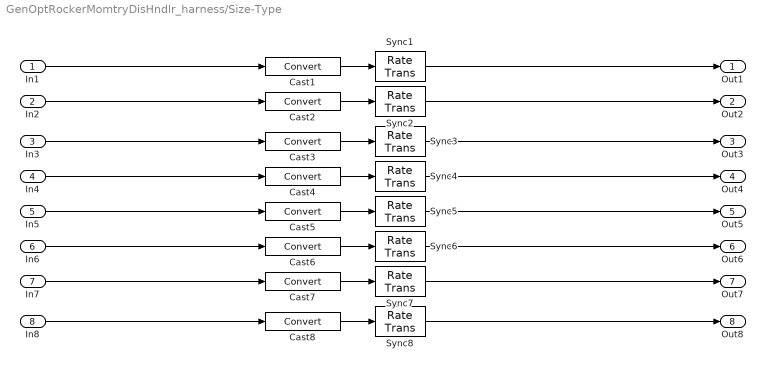
== system GenOptRockerMomtryDisHndlr_harness/Size-Type ==
  In1 : Inport
  In2 : Inport  Port=2
  In3 : Inport  Port=3
  In4 : Inport  Port=4
  In5 : Inport  Port=5
  In6 : Inport  Port=6
  In7 : Inport  Port=7
  In8 : Inport  Port=8
  Cast{1..8} (8 alike) : DataTypeConversion  RndMeth=Nearest  SaturateOnIntegerOverflow=on
  Sync{1..8} (8 alike) : RateTransition  OutPortSampleTimeOpt=Inherit  OutPortSampleTime=[0.01,0]
  Out1 : Outport
  Out2 : Outport  Port=2
  Out3 : Outport  Port=3
  Out4 : Outport  Port=4
  Out5 : Outport  Port=5
  Out6 : Outport  Port=6
  Out7 : Outport  Port=7
  Out8 : Outport  Port=8
  wires:
  In1/1 -> Cast1/1
  Cast1/1 -> Sync1/1
  Sync1/1 -> Out1/1
  In2/1 -> Cast2/1
  Cast2/1 -> Sync2/1
  Sync2/1 -> Out2/1
  In3/1 -> Cast3/1
  Cast3/1 -> Sync3/1
  Sync3/1 -> Out3/1
  In4/1 -> Cast4/1
  Cast4/1 -> Sync4/1
  Sync4/1 -> Out4/1
  In5/1 -> Cast5/1
  Cast5/1 -> Sync5/1
  Sync5/1 -> Out5/1
  In6/1 -> Cast6/1
  Cast6/1 -> Sync6/1
  Sync6/1 -> Out6/1
  In7/1 -> Cast7/1
  Cast7/1 -> Sync7/1
  Sync7/1 -> Out7/1
  In8/1 -> Cast8/1
  Cast8/1 -> Sync8/1
  Sync8/1 -> Out8/1

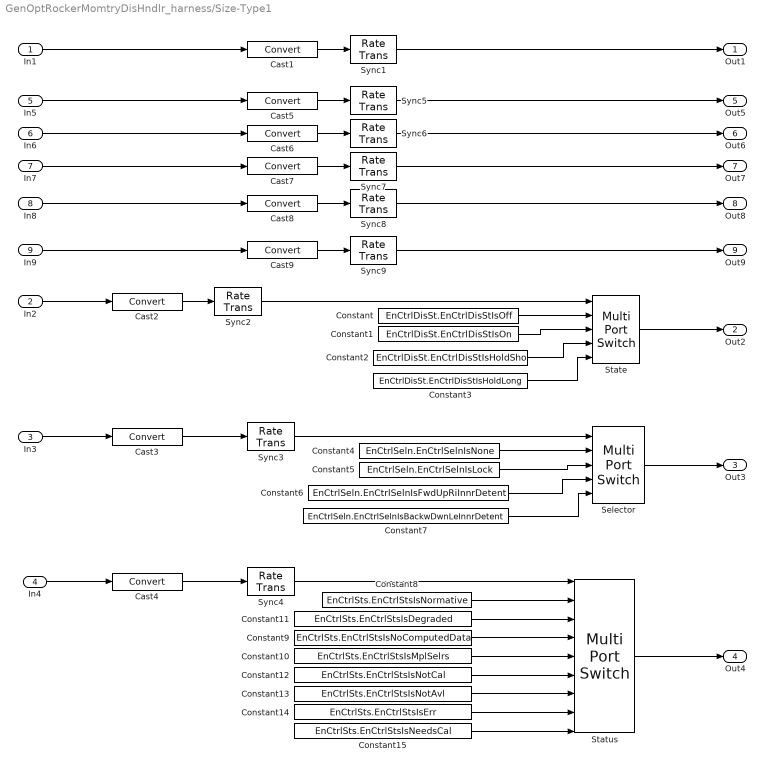
== system GenOptRockerMomtryDisHndlr_harness/Size-Type1 ==
  In1 : Inport
  In2 : Inport  Port=2
  In3 : Inport  Port=3
  In4 : Inport  Port=4
  In5 : Inport  Port=5
  In6 : Inport  Port=6
  In7 : Inport  Port=7
  In8 : Inport  Port=8
  In9 : Inport  Port=9
  " State" : MultiPortSwitch  DataPortOrder=Zero-based contiguous  Inputs=4  DataPortIndices={EnCtrlDisSt.EnCtrlDisStIsOff, EnCtrlDisSt.EnCtrlDisStIsOn, EnCtrlDisSt.EnCtrlDisStIsHoldSho, EnCtrlDisSt.EnCtrlDisStIsHoldLong}
  Cast{1..9} (9 alike) : DataTypeConversion  RndMeth=Nearest  SaturateOnIntegerOverflow=on
  Constant : Constant  Value=EnCtrlDisSt.EnCtrlDisStIsOff  OutDataTypeStr=Enum: EnCtrlDisSt
  Constant1 : Constant  Value=EnCtrlDisSt.EnCtrlDisStIsOn  OutDataTypeStr=Enum: EnCtrlDisSt
  Constant10 : Constant  Value=EnCtrlSts.EnCtrlStsIsMplSelrs  OutDataTypeStr=Enum: EnCtrlSts
  Constant11 : Constant  Value=EnCtrlSts.EnCtrlStsIsDegraded  OutDataTypeStr=Enum: EnCtrlSts
  Constant12 : Constant  Value=EnCtrlSts.EnCtrlStsIsNotCal  OutDataTypeStr=Enum: EnCtrlSts
  Constant13 : Constant  Value=EnCtrlSts.EnCtrlStsIsNotAvl  OutDataTypeStr=Enum: EnCtrlSts
  Constant14 : Constant  Value=EnCtrlSts.EnCtrlStsIsErr  OutDataTypeStr=Enum: EnCtrlSts
  Constant15 : Constant  Value=EnCtrlSts.EnCtrlStsIsNeedsCal  OutDataTypeStr=Enum: EnCtrlSts
  Constant2 : Constant  Value=EnCtrlDisSt.EnCtrlDisStIsHoldSho  OutDataTypeStr=Enum: EnCtrlDisSt
  Constant3 : Constant  Value=EnCtrlDisSt.EnCtrlDisStIsHoldLong  OutDataTypeStr=Enum: EnCtrlDisSt
  Constant4 : Constant  Value=EnCtrlSeln.EnCtrlSelnIsNone  OutDataTypeStr=Enum: EnCtrlSeln
  Constant5 : Constant  Value=EnCtrlSeln.EnCtrlSelnIsLock  OutDataTypeStr=Enum: EnCtrlSeln
  Constant6 : Constant  Value=EnCtrlSeln.EnCtrlSelnIsFwdUpRiInnrDetent  OutDataTypeStr=Enum: EnCtrlSeln
  Constant7 : Constant  Value=EnCtrlSeln.EnCtrlSelnIsBackwDwnLeInnrDetent  OutDataTypeStr=Enum: EnCtrlSeln
  Constant8 : Constant  Value=EnCtrlSts.EnCtrlStsIsNormative  OutDataTypeStr=Enum: EnCtrlSts
  Constant9 : Constant  Value=EnCtrlSts.EnCtrlStsIsNoComputedData  OutDataTypeStr=Enum: EnCtrlSts
  Selector : MultiPortSwitch  DataPortOrder=Zero-based contiguous  Inputs=4  DataPortIndices=[EnCtrlSeln.EnCtrlSelnIsNone, EnCtrlSeln.EnCtrlSelnIsLock, EnCtrlSeln.EnCtrlSelnIsFwdUpRiInnrDetent, EnCtrlSeln.EnCtrlSelnIsBackwDwnLeInnrDetent]
  Status : MultiPortSwitch  DataPortOrder=Zero-based contiguous  Inputs=8  DataPortIndices=[EnCtrlSts.EnCtrlStsIsNormative, EnCtrlSts.EnCtrlStsIsDegraded, EnCtrlSts.EnCtrlStsIsNoComputedData, EnCtrlSts.EnCtrlStsIsMplSelrs, EnCtrlSts.EnCtrlStsIsNotCal, EnCtrlSts.EnCtrlStsIsNotAvl, EnCtrlSts.EnCtrlStsIsErr, EnCtrlSts.EnCtrlStsIsNeedsCal]  OutDataTypeStr=Inherit: Inherit via back propagation
  Sync{1..9} (9 alike) : RateTransition  OutPortSampleTimeOpt=Inherit  OutPortSampleTime=[0.01,0]
  Out1 : Outport
  Out2 : Outport  Port=2
  Out3 : Outport  Port=3
  Out4 : Outport  Port=4
  Out5 : Outport  Port=5
  Out6 : Outport  Port=6
  Out7 : Outport  Port=7
  Out8 : Outport  Port=8
  Out9 : Outport  Port=9
  wires:
  In1/1 -> Cast1/1
  Cast1/1 -> Sync1/1
  Sync1/1 -> Out1/1
  In2/1 -> Cast2/1
  Cast2/1 -> Sync2/1
  In3/1 -> Cast3/1
  Cast3/1 -> Sync3/1
  In4/1 -> Cast4/1
  Cast4/1 -> Sync4/1
  In5/1 -> Cast5/1
  Cast5/1 -> Sync5/1
  Sync5/1 -> Out5/1
  In6/1 -> Cast6/1
  Cast6/1 -> Sync6/1
  Sync6/1 -> Out6/1
  In7/1 -> Cast7/1
  Cast7/1 -> Sync7/1
  Sync7/1 -> Out7/1
  In8/1 -> Cast8/1
  Cast8/1 -> Sync8/1
  Sync8/1 -> Out8/1
  Cast9/1 -> Sync9/1
  In9/1 -> Cast9/1
  Sync9/1 -> Out9/1
  Sync2/1 -> " State"/1
  " State"/1 -> Out2/1
  Constant/1 -> " State"/2
  Constant1/1 -> " State"/3
  Constant2/1 -> " State"/4
  Constant3/1 -> " State"/5
  Sync3/1 -> Selector/1
  Selector/1 -> Out3/1
  Constant4/1 -> Selector/2
  Constant5/1 -> Selector/3
  Constant6/1 -> Selector/4
  Constant7/1 -> Selector/5
  Sync4/1 -> Status/1
  Status/1 -> Out4/1
  Constant8/1 -> Status/2
  Constant11/1 -> Status/3
  Constant9/1 -> Status/4
  Constant10/1 -> Status/5
  Constant13/1 -> Status/7
  Constant12/1 -> Status/6
  Constant14/1 -> Status/8
  Constant15/1 -> Status/9
